simulink model "ALL_JP360_DBW_V6_5_1103"  (R2022a)
settings: Solver=FixedStepAuto  StartTime=0.0  StopTime=inf  FixedStep=0.01  RelTol=1e-3  EnableMultiTasking=on
model workspace (MAT data in the model file):
  g = 9.8
undefined symbols (not defined in the file or in its folder): canChannel, delta_v_p, IPM_Line_C0, IPM_Line_C1, IPM_Line_C2, IPM_Line_C3, M, M_p, MRR_ObjDistX, MRR_ObjDistY, MRR_ObjFusionCamID, MRR_ObjFusionSig, MRR_ObjID, MRR_ObjRelVelX, MRR_ObjRelVelY, MRR_ObjType, MRR_ObjUpdFlg, none, obj_vaild, untracktime, V, videoinput
libraries: canfdmsglib x230, canfdlib x76, slpidlib x24, simulink x18, dspstat3 x14, ctrlSharedLib x1, simulink_extras x1, imaqlib x1, realtime_pacer_lib x1, dspvision x1, visionsinks x1
(part 43 of 55)

== system ALL_JP360_DBW_V6_5_1103/MsgFromCAN/VR_ADCU_MsgFromCAN/VR_ADCU_IPM_Obj_04_0x653 ==
  VR_ADCU_IPM_Obj_04_0x653FromInData : Inport  OutDataTypeStr=Bus:CAN_FD_MESSAGE_BUS
  Bus Creator : BusCreator  Inputs=18  OutDataTypeStr=Bus:VR_ADCU_IPM_Obj_04_0x653  NonVirtualBus=on
  CAN FD Unpack : canfdmsglib/CAN FD Unpack  CANdbFile=HiFire_T360_P789_1R1V_Pri_Matrix_CAN_V2.3_20220810.dbc  MsgList=(none)  MsgName=IPM_Obj_04_0x653  ProtocolMode=CAN FD  MsgIDType=Standard (11-bit identifier)  MsgIdentifier=1619  MsgLength=32  SignalInfo={'IPM_ObjBlockCounter_04','13','11','BE','unsigned','Standard','0','1','0','0','2047';'IPM_ObjDistX_04','58','12','BE','unsigned','Standard','0','0.0625','0','0','254.9375';'IPM_ObjDistY_04','76','14','BE','unsigned','Standard','0','0.0078125','-64','-64','63.9922';'IPM_ObjID_04','16','8','BE','unsigned','Standard','0','1','0','0','255';'IPM_ObjRelAccelX_04','104','10','BE','unsigned','Standard','0','0.03125','-16','-16','15.9688';'IPM_ObjRelAccelY_04','126','10','BE','unsigned','Standard','0','0.03125','-16','-16','15.9688';'IPM_ObjRelVelX_04','95','13','BE','unsigned','Standard','0','0.03125','-128','-128','127.9688';'IPM_ObjRelVelY_04','98','13','BE','unsigned','Standard','0','0.03125','-128','-128','127.9688';'IPM_ObjType_04','54','4','BE','unsigned','Standard','0','1','0','0','15';'IPM_Obj_04_Checksum','248','16','BE','unsigned','Standard','0','1','0','0','65535';'IPM_Obj_04_MsgCounter','232','4','BE','unsigned','Standard','0','1','0','0','15';'IPM_Object_Age_04','37','11','BE','unsigned','Standard','0','1','0','0','2047';'IPM_Object_Existence_Probability_04','42','6','BE','unsigned','Standard','0','2','0','0','100';'IPM_Object_Heading_04','132','10','BE','unsigned','Standard','0','0.01','-3.14','-3.14','3.14';'IPM_Object_Height_04','167','9','BE','unsigned','Standard','0','0.01','0','0','5.11';'IPM_Object_Length_04','139','9','BE','unsigned','Standard','0','0.05','0','0','25.5';'IPM_Object_Motion_Status_04','161','3','BE','unsigned','Standard','0','1','0','0','7';'IPM_Object_Width_04','144','11','BE','unsigned','Standard','0','0.01','0','0','12'}  IDPort=off  TimestampPort=off  ErrorPort=off  RemotePort=off  LengthPort=off  StatusPort=off  BRSPort=off  ESIPort=off  DLCPort=off  ApplyMinMax=off
      settings: SourceProductBaseCode=ME,XP,VN  DataFormat=CANdb specified signals
  Data Type Conversion1 : DataTypeConversion  OutDataTypeStr=int16  SaturateOnIntegerOverflow=off  RndMeth=Floor
  Data Type Conversion10 : DataTypeConversion  OutDataTypeStr=uint16  SaturateOnIntegerOverflow=off  RndMeth=Floor
  Data Type Conversion{9,11,13,17} (4 alike) : DataTypeConversion  OutDataTypeStr=int8  SaturateOnIntegerOverflow=off  RndMeth=Floor
  Data Type Conversion12 : DataTypeConversion  OutDataTypeStr=int16  SaturateOnIntegerOverflow=off  RndMeth=Floor
  Data Type Conversion{2..3,5..8,14..16,18} (10 alike) : DataTypeConversion  OutDataTypeStr=single  SaturateOnIntegerOverflow=off  RndMeth=Floor
  Data Type Conversion4 : DataTypeConversion  OutDataTypeStr=uint8  SaturateOnIntegerOverflow=off  RndMeth=Floor
  VR_ADCU_IPM_Obj_04_0x653FromOutData : Outport  OutDataTypeStr=Bus:VR_ADCU_IPM_Obj_04_0x653
  wires:
  CAN FD Unpack/1 -> Data Type Conversion1/1
  CAN FD Unpack/2 -> Data Type Conversion2/1
  CAN FD Unpack/3 -> Data Type Conversion3/1
  CAN FD Unpack/4 -> Data Type Conversion4/1
  CAN FD Unpack/5 -> Data Type Conversion5/1
  CAN FD Unpack/6 -> Data Type Conversion6/1
  CAN FD Unpack/7 -> Data Type Conversion7/1
  CAN FD Unpack/8 -> Data Type Conversion8/1
  CAN FD Unpack/9 -> Data Type Conversion9/1
  CAN FD Unpack/10 -> Data Type Conversion10/1
  CAN FD Unpack/11 -> Data Type Conversion11/1
  CAN FD Unpack/12 -> Data Type Conversion12/1
  CAN FD Unpack/13 -> Data Type Conversion13/1
  CAN FD Unpack/14 -> Data Type Conversion14/1
  CAN FD Unpack/15 -> Data Type Conversion15/1
  CAN FD Unpack/16 -> Data Type Conversion16/1
  CAN FD Unpack/17 -> Data Type Conversion17/1
  CAN FD Unpack/18 -> Data Type Conversion18/1
  Data Type Conversion1/1 -> Bus Creator/1  "IPM_ObjBlockCounter_04"
  Data Type Conversion2/1 -> Bus Creator/2  "IPM_ObjDistX_04"
  Data Type Conversion3/1 -> Bus Creator/3  "IPM_ObjDistY_04"
  Data Type Conversion4/1 -> Bus Creator/4  "IPM_ObjID_04"
  Data Type Conversion5/1 -> Bus Creator/5  "IPM_ObjRelAccelX_04"
  Data Type Conversion6/1 -> Bus Creator/6  "IPM_ObjRelAccelY_04"
  Data Type Conversion7/1 -> Bus Creator/7  "IPM_ObjRelVelX_04"
  Data Type Conversion8/1 -> Bus Creator/8  "IPM_ObjRelVelY_04"
  Data Type Conversion9/1 -> Bus Creator/9  "IPM_ObjType_04"
  Data Type Conversion10/1 -> Bus Creator/10  "IPM_Obj_04_Checksum"
  Data Type Conversion11/1 -> Bus Creator/11  "IPM_Obj_04_MsgCounter"
  Data Type Conversion12/1 -> Bus Creator/12  "IPM_Object_Age_04"
  Data Type Conversion13/1 -> Bus Creator/13  "IPM_Object_Existence_Probability_04"
  Data Type Conversion14/1 -> Bus Creator/14  "IPM_Object_Heading_04"
  Data Type Conversion15/1 -> Bus Creator/15  "IPM_Object_Height_04"
  Data Type Conversion16/1 -> Bus Creator/16  "IPM_Object_Length_04"
  Data Type Conversion17/1 -> Bus Creator/17  "IPM_Object_Motion_Status_04"
  Data Type Conversion18/1 -> Bus Creator/18  "IPM_Object_Width_04"
  Bus Creator/1 -> VR_ADCU_IPM_Obj_04_0x653FromOutData/1  "VR_ADCU_IPM_Obj_04_0x653FromOutData"
  VR_ADCU_IPM_Obj_04_0x653FromInData/1 -> CAN FD Unpack/1  "VR_ADCU_IPM_Obj_04_0x653FromInData"

== system ALL_JP360_DBW_V6_5_1103/MsgFromCAN/VR_ADCU_MsgFromCAN/VR_ADCU_IPM_Obj_05_0x654 ==
  VR_ADCU_IPM_Obj_05_0x654FromInData : Inport  OutDataTypeStr=Bus:CAN_FD_MESSAGE_BUS
  Bus Creator : BusCreator  Inputs=18  OutDataTypeStr=Bus:VR_ADCU_IPM_Obj_05_0x654  NonVirtualBus=on
  CAN FD Unpack : canfdmsglib/CAN FD Unpack  CANdbFile=HiFire_T360_P789_1R1V_Pri_Matrix_CAN_V2.3_20220810.dbc  MsgList=(none)  MsgName=IPM_Obj_05_0x654  ProtocolMode=CAN FD  MsgIDType=Standard (11-bit identifier)  MsgIdentifier=1620  MsgLength=32  SignalInfo={'IPM_ObjBlockCounter_05','13','11','BE','unsigned','Standard','0','1','0','0','2047';'IPM_ObjDistX_05','58','12','BE','unsigned','Standard','0','0.0625','0','0','254.9375';'IPM_ObjDistY_05','76','14','BE','unsigned','Standard','0','0.0078125','-64','-64','63.9922';'IPM_ObjID_05','16','8','BE','unsigned','Standard','0','1','0','0','255';'IPM_ObjRelAccelX_05','104','10','BE','unsigned','Standard','0','0.03125','-16','-16','15.9688';'IPM_ObjRelAccelY_05','126','10','BE','unsigned','Standard','0','0.03125','-16','-16','15.9688';'IPM_ObjRelVelX_05','95','13','BE','unsigned','Standard','0','0.03125','-128','-128','127.9688';'IPM_ObjRelVelY_05','98','13','BE','unsigned','Standard','0','0.03125','-128','-128','127.9688';'IPM_ObjType_05','54','4','BE','unsigned','Standard','0','1','0','0','15';'IPM_Obj_05_Checksum','248','16','BE','unsigned','Standard','0','1','0','0','65535';'IPM_Obj_05_MsgCounter','232','4','BE','unsigned','Standard','0','1','0','0','15';'IPM_Object_Age_05','37','11','BE','unsigned','Standard','0','1','0','0','2047';'IPM_Object_Existence_Probability_05','42','6','BE','unsigned','Standard','0','2','0','0','100';'IPM_Object_Heading_05','132','10','BE','unsigned','Standard','0','0.01','-3.14','-3.14','3.14';'IPM_Object_Height_05','167','9','BE','unsigned','Standard','0','0.01','0','0','5.11';'IPM_Object_Length_05','139','9','BE','unsigned','Standard','0','0.05','0','0','25.5';'IPM_Object_Motion_Status_05','161','3','BE','unsigned','Standard','0','1','0','0','7';'IPM_Object_Width_05','144','11','BE','unsigned','Standard','0','0.01','0','0','12'}  IDPort=off  TimestampPort=off  ErrorPort=off  RemotePort=off  LengthPort=off  StatusPort=off  BRSPort=off  ESIPort=off  DLCPort=off  ApplyMinMax=off
      settings: SourceProductBaseCode=ME,XP,VN  DataFormat=CANdb specified signals
  Data Type Conversion1 : DataTypeConversion  OutDataTypeStr=int16  SaturateOnIntegerOverflow=off  RndMeth=Floor
  Data Type Conversion10 : DataTypeConversion  OutDataTypeStr=uint16  SaturateOnIntegerOverflow=off  RndMeth=Floor
  Data Type Conversion{9,11,13,17} (4 alike) : DataTypeConversion  OutDataTypeStr=int8  SaturateOnIntegerOverflow=off  RndMeth=Floor
  Data Type Conversion12 : DataTypeConversion  OutDataTypeStr=int16  SaturateOnIntegerOverflow=off  RndMeth=Floor
  Data Type Conversion{2..3,5..8,14..16,18} (10 alike) : DataTypeConversion  OutDataTypeStr=single  SaturateOnIntegerOverflow=off  RndMeth=Floor
  Data Type Conversion4 : DataTypeConversion  OutDataTypeStr=uint8  SaturateOnIntegerOverflow=off  RndMeth=Floor
  VR_ADCU_IPM_Obj_05_0x654FromOutData : Outport  OutDataTypeStr=Bus:VR_ADCU_IPM_Obj_05_0x654
  wires:
  CAN FD Unpack/1 -> Data Type Conversion1/1
  CAN FD Unpack/2 -> Data Type Conversion2/1
  CAN FD Unpack/3 -> Data Type Conversion3/1
  CAN FD Unpack/4 -> Data Type Conversion4/1
  CAN FD Unpack/5 -> Data Type Conversion5/1
  CAN FD Unpack/6 -> Data Type Conversion6/1
  CAN FD Unpack/7 -> Data Type Conversion7/1
  CAN FD Unpack/8 -> Data Type Conversion8/1
  CAN FD Unpack/9 -> Data Type Conversion9/1
  CAN FD Unpack/10 -> Data Type Conversion10/1
  CAN FD Unpack/11 -> Data Type Conversion11/1
  CAN FD Unpack/12 -> Data Type Conversion12/1
  CAN FD Unpack/13 -> Data Type Conversion13/1
  CAN FD Unpack/14 -> Data Type Conversion14/1
  CAN FD Unpack/15 -> Data Type Conversion15/1
  CAN FD Unpack/16 -> Data Type Conversion16/1
  CAN FD Unpack/17 -> Data Type Conversion17/1
  CAN FD Unpack/18 -> Data Type Conversion18/1
  Data Type Conversion1/1 -> Bus Creator/1  "IPM_ObjBlockCounter_05"
  Data Type Conversion2/1 -> Bus Creator/2  "IPM_ObjDistX_05"
  Data Type Conversion3/1 -> Bus Creator/3  "IPM_ObjDistY_05"
  Data Type Conversion4/1 -> Bus Creator/4  "IPM_ObjID_05"
  Data Type Conversion5/1 -> Bus Creator/5  "IPM_ObjRelAccelX_05"
  Data Type Conversion6/1 -> Bus Creator/6  "IPM_ObjRelAccelY_05"
  Data Type Conversion7/1 -> Bus Creator/7  "IPM_ObjRelVelX_05"
  Data Type Conversion8/1 -> Bus Creator/8  "IPM_ObjRelVelY_05"
  Data Type Conversion9/1 -> Bus Creator/9  "IPM_ObjType_05"
  Data Type Conversion10/1 -> Bus Creator/10  "IPM_Obj_05_Checksum"
  Data Type Conversion11/1 -> Bus Creator/11  "IPM_Obj_05_MsgCounter"
  Data Type Conversion12/1 -> Bus Creator/12  "IPM_Object_Age_05"
  Data Type Conversion13/1 -> Bus Creator/13  "IPM_Object_Existence_Probability_05"
  Data Type Conversion14/1 -> Bus Creator/14  "IPM_Object_Heading_05"
  Data Type Conversion15/1 -> Bus Creator/15  "IPM_Object_Height_05"
  Data Type Conversion16/1 -> Bus Creator/16  "IPM_Object_Length_05"
  Data Type Conversion17/1 -> Bus Creator/17  "IPM_Object_Motion_Status_05"
  Data Type Conversion18/1 -> Bus Creator/18  "IPM_Object_Width_05"
  Bus Creator/1 -> VR_ADCU_IPM_Obj_05_0x654FromOutData/1  "VR_ADCU_IPM_Obj_05_0x654FromOutData"
  VR_ADCU_IPM_Obj_05_0x654FromInData/1 -> CAN FD Unpack/1  "VR_ADCU_IPM_Obj_05_0x654FromInData"

== system ALL_JP360_DBW_V6_5_1103/MsgFromCAN/VR_ADCU_MsgFromCAN/VR_ADCU_IPM_Obj_06_0x655 ==
  VR_ADCU_IPM_Obj_06_0x655FromInData : Inport  OutDataTypeStr=Bus:CAN_FD_MESSAGE_BUS
  Bus Creator : BusCreator  Inputs=18  OutDataTypeStr=Bus:VR_ADCU_IPM_Obj_06_0x655  NonVirtualBus=on
  CAN FD Unpack : canfdmsglib/CAN FD Unpack  CANdbFile=HiFire_T360_P789_1R1V_Pri_Matrix_CAN_V2.3_20220810.dbc  MsgList=(none)  MsgName=IPM_Obj_06_0x655  ProtocolMode=CAN FD  MsgIDType=Standard (11-bit identifier)  MsgIdentifier=1621  MsgLength=32  SignalInfo={'IPM_ObjBlockCounter_06','13','11','BE','unsigned','Standard','0','1','0','0','2047';'IPM_ObjDistX_06','58','12','BE','unsigned','Standard','0','0.0625','0','0','254.9375';'IPM_ObjDistY_06','76','14','BE','unsigned','Standard','0','0.0078125','-64','-64','63.9922';'IPM_ObjID_06','16','8','BE','unsigned','Standard','0','1','0','0','255';'IPM_ObjRelAccelX_06','104','10','BE','unsigned','Standard','0','0.03125','-16','-16','15.9688';'IPM_ObjRelAccelY_06','126','10','BE','unsigned','Standard','0','0.03125','-16','-16','15.9688';'IPM_ObjRelVelX_06','95','13','BE','unsigned','Standard','0','0.03125','-128','-128','127.9688';'IPM_ObjRelVelY_06','98','13','BE','unsigned','Standard','0','0.03125','-128','-128','127.9688';'IPM_ObjType_06','54','4','BE','unsigned','Standard','0','1','0','0','15';'IPM_Obj_06_Checksum','248','16','BE','unsigned','Standard','0','1','0','0','65535';'IPM_Obj_06_MsgCounter','232','4','BE','unsigned','Standard','0','1','0','0','15';'IPM_Object_Age_06','37','11','BE','unsigned','Standard','0','1','0','0','2047';'IPM_Object_Existence_Probability_06','42','6','BE','unsigned','Standard','0','2','0','0','100';'IPM_Object_Heading_06','132','10','BE','unsigned','Standard','0','0.01','-3.14','-3.14','3.14';'IPM_Object_Height_06','167','9','BE','unsigned','Standard','0','0.01','0','0','5.11';'IPM_Object_Length_06','139','9','BE','unsigned','Standard','0','0.05','0','0','25.5';'IPM_Object_Motion_Status_06','161','3','BE','unsigned','Standard','0','1','0','0','7';'IPM_Object_Width_06','144','11','BE','unsigned','Standard','0','0.01','0','0','12'}  IDPort=off  TimestampPort=off  ErrorPort=off  RemotePort=off  LengthPort=off  StatusPort=off  BRSPort=off  ESIPort=off  DLCPort=off  ApplyMinMax=off
      settings: SourceProductBaseCode=ME,XP,VN  DataFormat=CANdb specified signals
  Data Type Conversion1 : DataTypeConversion  OutDataTypeStr=int16  SaturateOnIntegerOverflow=off  RndMeth=Floor
  Data Type Conversion10 : DataTypeConversion  OutDataTypeStr=uint16  SaturateOnIntegerOverflow=off  RndMeth=Floor
  Data Type Conversion{9,11,13,17} (4 alike) : DataTypeConversion  OutDataTypeStr=int8  SaturateOnIntegerOverflow=off  RndMeth=Floor
  Data Type Conversion12 : DataTypeConversion  OutDataTypeStr=int16  SaturateOnIntegerOverflow=off  RndMeth=Floor
  Data Type Conversion{2..3,5..8,14..16,18} (10 alike) : DataTypeConversion  OutDataTypeStr=single  SaturateOnIntegerOverflow=off  RndMeth=Floor
  Data Type Conversion4 : DataTypeConversion  OutDataTypeStr=uint8  SaturateOnIntegerOverflow=off  RndMeth=Floor
  VR_ADCU_IPM_Obj_06_0x655FromOutData : Outport  OutDataTypeStr=Bus:VR_ADCU_IPM_Obj_06_0x655
  wires:
  CAN FD Unpack/1 -> Data Type Conversion1/1
  CAN FD Unpack/2 -> Data Type Conversion2/1
  CAN FD Unpack/3 -> Data Type Conversion3/1
  CAN FD Unpack/4 -> Data Type Conversion4/1
  CAN FD Unpack/5 -> Data Type Conversion5/1
  CAN FD Unpack/6 -> Data Type Conversion6/1
  CAN FD Unpack/7 -> Data Type Conversion7/1
  CAN FD Unpack/8 -> Data Type Conversion8/1
  CAN FD Unpack/9 -> Data Type Conversion9/1
  CAN FD Unpack/10 -> Data Type Conversion10/1
  CAN FD Unpack/11 -> Data Type Conversion11/1
  CAN FD Unpack/12 -> Data Type Conversion12/1
  CAN FD Unpack/13 -> Data Type Conversion13/1
  CAN FD Unpack/14 -> Data Type Conversion14/1
  CAN FD Unpack/15 -> Data Type Conversion15/1
  CAN FD Unpack/16 -> Data Type Conversion16/1
  CAN FD Unpack/17 -> Data Type Conversion17/1
  CAN FD Unpack/18 -> Data Type Conversion18/1
  Data Type Conversion1/1 -> Bus Creator/1  "IPM_ObjBlockCounter_06"
  Data Type Conversion2/1 -> Bus Creator/2  "IPM_ObjDistX_06"
  Data Type Conversion3/1 -> Bus Creator/3  "IPM_ObjDistY_06"
  Data Type Conversion4/1 -> Bus Creator/4  "IPM_ObjID_06"
  Data Type Conversion5/1 -> Bus Creator/5  "IPM_ObjRelAccelX_06"
  Data Type Conversion6/1 -> Bus Creator/6  "IPM_ObjRelAccelY_06"
  Data Type Conversion7/1 -> Bus Creator/7  "IPM_ObjRelVelX_06"
  Data Type Conversion8/1 -> Bus Creator/8  "IPM_ObjRelVelY_06"
  Data Type Conversion9/1 -> Bus Creator/9  "IPM_ObjType_06"
  Data Type Conversion10/1 -> Bus Creator/10  "IPM_Obj_06_Checksum"
  Data Type Conversion11/1 -> Bus Creator/11  "IPM_Obj_06_MsgCounter"
  Data Type Conversion12/1 -> Bus Creator/12  "IPM_Object_Age_06"
  Data Type Conversion13/1 -> Bus Creator/13  "IPM_Object_Existence_Probability_06"
  Data Type Conversion14/1 -> Bus Creator/14  "IPM_Object_Heading_06"
  Data Type Conversion15/1 -> Bus Creator/15  "IPM_Object_Height_06"
  Data Type Conversion16/1 -> Bus Creator/16  "IPM_Object_Length_06"
  Data Type Conversion17/1 -> Bus Creator/17  "IPM_Object_Motion_Status_06"
  Data Type Conversion18/1 -> Bus Creator/18  "IPM_Object_Width_06"
  Bus Creator/1 -> VR_ADCU_IPM_Obj_06_0x655FromOutData/1  "VR_ADCU_IPM_Obj_06_0x655FromOutData"
  VR_ADCU_IPM_Obj_06_0x655FromInData/1 -> CAN FD Unpack/1  "VR_ADCU_IPM_Obj_06_0x655FromInData"

== system ALL_JP360_DBW_V6_5_1103/MsgFromCAN/VR_ADCU_MsgFromCAN/VR_ADCU_IPM_Obj_07_0x656 ==
  VR_ADCU_IPM_Obj_07_0x656FromInData : Inport  OutDataTypeStr=Bus:CAN_FD_MESSAGE_BUS
  Bus Creator : BusCreator  Inputs=18  OutDataTypeStr=Bus:VR_ADCU_IPM_Obj_07_0x656  NonVirtualBus=on
  CAN FD Unpack : canfdmsglib/CAN FD Unpack  CANdbFile=HiFire_T360_P789_1R1V_Pri_Matrix_CAN_V2.3_20220810.dbc  MsgList=(none)  MsgName=IPM_Obj_07_0x656  ProtocolMode=CAN FD  MsgIDType=Standard (11-bit identifier)  MsgIdentifier=1622  MsgLength=32  SignalInfo={'IPM_ObjBlockCounter_07','13','11','BE','unsigned','Standard','0','1','0','0','2047';'IPM_ObjDistX_07','58','12','BE','unsigned','Standard','0','0.0625','0','0','254.9375';'IPM_ObjDistY_07','76','14','BE','unsigned','Standard','0','0.0078125','-64','-64','63.9922';'IPM_ObjID_07','16','8','BE','unsigned','Standard','0','1','0','0','255';'IPM_ObjRelAccelX_07','104','10','BE','unsigned','Standard','0','0.03125','-16','-16','15.9688';'IPM_ObjRelAccelY_07','126','10','BE','unsigned','Standard','0','0.03125','-16','-16','15.9688';'IPM_ObjRelVelX_07','95','13','BE','unsigned','Standard','0','0.03125','-128','-128','127.9688';'IPM_ObjRelVelY_07','98','13','BE','unsigned','Standard','0','0.03125','-128','-128','127.9688';'IPM_ObjType_07','54','4','BE','unsigned','Standard','0','1','0','0','15';'IPM_Obj_07_Checksum','248','16','BE','unsigned','Standard','0','1','0','0','65535';'IPM_Obj_07_MsgCounter','232','4','BE','unsigned','Standard','0','1','0','0','15';'IPM_Object_Age_07','37','11','BE','unsigned','Standard','0','1','0','0','2047';'IPM_Object_Existence_Probability_07','42','6','BE','unsigned','Standard','0','2','0','0','100';'IPM_Object_Heading_07','132','10','BE','unsigned','Standard','0','0.01','-3.14','-3.14','3.14';'IPM_Object_Height_07','167','9','BE','unsigned','Standard','0','0.01','0','0','5.11';'IPM_Object_Length_07','139','9','BE','unsigned','Standard','0','0.05','0','0','25.5';'IPM_Object_Motion_Status_07','161','3','BE','unsigned','Standard','0','1','0','0','7';'IPM_Object_Width_07','144','11','BE','unsigned','Standard','0','0.01','0','0','12'}  IDPort=off  TimestampPort=off  ErrorPort=off  RemotePort=off  LengthPort=off  StatusPort=off  BRSPort=off  ESIPort=off  DLCPort=off  ApplyMinMax=off
      settings: SourceProductBaseCode=ME,XP,VN  DataFormat=CANdb specified signals
  Data Type Conversion1 : DataTypeConversion  OutDataTypeStr=int16  SaturateOnIntegerOverflow=off  RndMeth=Floor
  Data Type Conversion10 : DataTypeConversion  OutDataTypeStr=uint16  SaturateOnIntegerOverflow=off  RndMeth=Floor
  Data Type Conversion{9,11,13,17} (4 alike) : DataTypeConversion  OutDataTypeStr=int8  SaturateOnIntegerOverflow=off  RndMeth=Floor
  Data Type Conversion12 : DataTypeConversion  OutDataTypeStr=int16  SaturateOnIntegerOverflow=off  RndMeth=Floor
  Data Type Conversion{2..3,5..8,14..16,18} (10 alike) : DataTypeConversion  OutDataTypeStr=single  SaturateOnIntegerOverflow=off  RndMeth=Floor
  Data Type Conversion4 : DataTypeConversion  OutDataTypeStr=uint8  SaturateOnIntegerOverflow=off  RndMeth=Floor
  VR_ADCU_IPM_Obj_07_0x656FromOutData : Outport  OutDataTypeStr=Bus:VR_ADCU_IPM_Obj_07_0x656
  wires:
  CAN FD Unpack/1 -> Data Type Conversion1/1
  CAN FD Unpack/2 -> Data Type Conversion2/1
  CAN FD Unpack/3 -> Data Type Conversion3/1
  CAN FD Unpack/4 -> Data Type Conversion4/1
  CAN FD Unpack/5 -> Data Type Conversion5/1
  CAN FD Unpack/6 -> Data Type Conversion6/1
  CAN FD Unpack/7 -> Data Type Conversion7/1
  CAN FD Unpack/8 -> Data Type Conversion8/1
  CAN FD Unpack/9 -> Data Type Conversion9/1
  CAN FD Unpack/10 -> Data Type Conversion10/1
  CAN FD Unpack/11 -> Data Type Conversion11/1
  CAN FD Unpack/12 -> Data Type Conversion12/1
  CAN FD Unpack/13 -> Data Type Conversion13/1
  CAN FD Unpack/14 -> Data Type Conversion14/1
  CAN FD Unpack/15 -> Data Type Conversion15/1
  CAN FD Unpack/16 -> Data Type Conversion16/1
  CAN FD Unpack/17 -> Data Type Conversion17/1
  CAN FD Unpack/18 -> Data Type Conversion18/1
  Data Type Conversion1/1 -> Bus Creator/1  "IPM_ObjBlockCounter_07"
  Data Type Conversion2/1 -> Bus Creator/2  "IPM_ObjDistX_07"
  Data Type Conversion3/1 -> Bus Creator/3  "IPM_ObjDistY_07"
  Data Type Conversion4/1 -> Bus Creator/4  "IPM_ObjID_07"
  Data Type Conversion5/1 -> Bus Creator/5  "IPM_ObjRelAccelX_07"
  Data Type Conversion6/1 -> Bus Creator/6  "IPM_ObjRelAccelY_07"
  Data Type Conversion7/1 -> Bus Creator/7  "IPM_ObjRelVelX_07"
  Data Type Conversion8/1 -> Bus Creator/8  "IPM_ObjRelVelY_07"
  Data Type Conversion9/1 -> Bus Creator/9  "IPM_ObjType_07"
  Data Type Conversion10/1 -> Bus Creator/10  "IPM_Obj_07_Checksum"
  Data Type Conversion11/1 -> Bus Creator/11  "IPM_Obj_07_MsgCounter"
  Data Type Conversion12/1 -> Bus Creator/12  "IPM_Object_Age_07"
  Data Type Conversion13/1 -> Bus Creator/13  "IPM_Object_Existence_Probability_07"
  Data Type Conversion14/1 -> Bus Creator/14  "IPM_Object_Heading_07"
  Data Type Conversion15/1 -> Bus Creator/15  "IPM_Object_Height_07"
  Data Type Conversion16/1 -> Bus Creator/16  "IPM_Object_Length_07"
  Data Type Conversion17/1 -> Bus Creator/17  "IPM_Object_Motion_Status_07"
  Data Type Conversion18/1 -> Bus Creator/18  "IPM_Object_Width_07"
  Bus Creator/1 -> VR_ADCU_IPM_Obj_07_0x656FromOutData/1  "VR_ADCU_IPM_Obj_07_0x656FromOutData"
  VR_ADCU_IPM_Obj_07_0x656FromInData/1 -> CAN FD Unpack/1  "VR_ADCU_IPM_Obj_07_0x656FromInData"

== system ALL_JP360_DBW_V6_5_1103/MsgFromCAN/VR_ADCU_MsgFromCAN/VR_ADCU_IPM_Obj_08_0x657 ==
  VR_ADCU_IPM_Obj_08_0x657FromInData : Inport  OutDataTypeStr=Bus:CAN_FD_MESSAGE_BUS
  Bus Creator : BusCreator  Inputs=18  OutDataTypeStr=Bus:VR_ADCU_IPM_Obj_08_0x657  NonVirtualBus=on
  CAN FD Unpack : canfdmsglib/CAN FD Unpack  CANdbFile=HiFire_T360_P789_1R1V_Pri_Matrix_CAN_V2.3_20220810.dbc  MsgList=(none)  MsgName=IPM_Obj_08_0x657  ProtocolMode=CAN FD  MsgIDType=Standard (11-bit identifier)  MsgIdentifier=1623  MsgLength=32  SignalInfo={'IPM_ObjBlockCounter_08','13','11','BE','unsigned','Standard','0','1','0','0','2047';'IPM_ObjDistX_08','58','12','BE','unsigned','Standard','0','0.0625','0','0','254.9375';'IPM_ObjDistY_08','76','14','BE','unsigned','Standard','0','0.0078125','-64','-64','63.9922';'IPM_ObjID_08','16','8','BE','unsigned','Standard','0','1','0','0','255';'IPM_ObjRelAccelX_08','104','10','BE','unsigned','Standard','0','0.03125','-16','-16','15.9688';'IPM_ObjRelAccelY_08','126','10','BE','unsigned','Standard','0','0.03125','-16','-16','15.9688';'IPM_ObjRelVelX_08','95','13','BE','unsigned','Standard','0','0.03125','-128','-128','127.9688';'IPM_ObjRelVelY_08','98','13','BE','unsigned','Standard','0','0.03125','-128','-128','127.9688';'IPM_ObjType_08','54','4','BE','unsigned','Standard','0','1','0','0','15';'IPM_Obj_08_Checksum','248','16','BE','unsigned','Standard','0','1','0','0','65535';'IPM_Obj_08_MsgCounter','232','4','BE','unsigned','Standard','0','1','0','0','15';'IPM_Object_Age_08','37','11','BE','unsigned','Standard','0','1','0','0','2047';'IPM_Object_Existence_Probability_08','42','6','BE','unsigned','Standard','0','2','0','0','100';'IPM_Object_Heading_08','132','10','BE','unsigned','Standard','0','0.01','-3.14','-3.14','3.14';'IPM_Object_Height_08','167','9','BE','unsigned','Standard','0','0.01','0','0','5.11';'IPM_Object_Length_08','139','9','BE','unsigned','Standard','0','0.05','0','0','25.5';'IPM_Object_Motion_Status_08','161','3','BE','unsigned','Standard','0','1','0','0','7';'IPM_Object_Width_08','144','11','BE','unsigned','Standard','0','0.01','0','0','12'}  IDPort=off  TimestampPort=off  ErrorPort=off  RemotePort=off  LengthPort=off  StatusPort=off  BRSPort=off  ESIPort=off  DLCPort=off  ApplyMinMax=off
      settings: SourceProductBaseCode=ME,XP,VN  DataFormat=CANdb specified signals
  Data Type Conversion1 : DataTypeConversion  OutDataTypeStr=int16  SaturateOnIntegerOverflow=off  RndMeth=Floor
  Data Type Conversion10 : DataTypeConversion  OutDataTypeStr=uint16  SaturateOnIntegerOverflow=off  RndMeth=Floor
  Data Type Conversion{9,11,13,17} (4 alike) : DataTypeConversion  OutDataTypeStr=int8  SaturateOnIntegerOverflow=off  RndMeth=Floor
  Data Type Conversion12 : DataTypeConversion  OutDataTypeStr=int16  SaturateOnIntegerOverflow=off  RndMeth=Floor
  Data Type Conversion{2..3,5..8,14..16,18} (10 alike) : DataTypeConversion  OutDataTypeStr=single  SaturateOnIntegerOverflow=off  RndMeth=Floor
  Data Type Conversion4 : DataTypeConversion  OutDataTypeStr=uint8  SaturateOnIntegerOverflow=off  RndMeth=Floor
  VR_ADCU_IPM_Obj_08_0x657FromOutData : Outport  OutDataTypeStr=Bus:VR_ADCU_IPM_Obj_08_0x657
  wires:
  CAN FD Unpack/1 -> Data Type Conversion1/1
  CAN FD Unpack/2 -> Data Type Conversion2/1
  CAN FD Unpack/3 -> Data Type Conversion3/1
  CAN FD Unpack/4 -> Data Type Conversion4/1
  CAN FD Unpack/5 -> Data Type Conversion5/1
  CAN FD Unpack/6 -> Data Type Conversion6/1
  CAN FD Unpack/7 -> Data Type Conversion7/1
  CAN FD Unpack/8 -> Data Type Conversion8/1
  CAN FD Unpack/9 -> Data Type Conversion9/1
  CAN FD Unpack/10 -> Data Type Conversion10/1
  CAN FD Unpack/11 -> Data Type Conversion11/1
  CAN FD Unpack/12 -> Data Type Conversion12/1
  CAN FD Unpack/13 -> Data Type Conversion13/1
  CAN FD Unpack/14 -> Data Type Conversion14/1
  CAN FD Unpack/15 -> Data Type Conversion15/1
  CAN FD Unpack/16 -> Data Type Conversion16/1
  CAN FD Unpack/17 -> Data Type Conversion17/1
  CAN FD Unpack/18 -> Data Type Conversion18/1
  Data Type Conversion1/1 -> Bus Creator/1  "IPM_ObjBlockCounter_08"
  Data Type Conversion2/1 -> Bus Creator/2  "IPM_ObjDistX_08"
  Data Type Conversion3/1 -> Bus Creator/3  "IPM_ObjDistY_08"
  Data Type Conversion4/1 -> Bus Creator/4  "IPM_ObjID_08"
  Data Type Conversion5/1 -> Bus Creator/5  "IPM_ObjRelAccelX_08"
  Data Type Conversion6/1 -> Bus Creator/6  "IPM_ObjRelAccelY_08"
  Data Type Conversion7/1 -> Bus Creator/7  "IPM_ObjRelVelX_08"
  Data Type Conversion8/1 -> Bus Creator/8  "IPM_ObjRelVelY_08"
  Data Type Conversion9/1 -> Bus Creator/9  "IPM_ObjType_08"
  Data Type Conversion10/1 -> Bus Creator/10  "IPM_Obj_08_Checksum"
  Data Type Conversion11/1 -> Bus Creator/11  "IPM_Obj_08_MsgCounter"
  Data Type Conversion12/1 -> Bus Creator/12  "IPM_Object_Age_08"
  Data Type Conversion13/1 -> Bus Creator/13  "IPM_Object_Existence_Probability_08"
  Data Type Conversion14/1 -> Bus Creator/14  "IPM_Object_Heading_08"
  Data Type Conversion15/1 -> Bus Creator/15  "IPM_Object_Height_08"
  Data Type Conversion16/1 -> Bus Creator/16  "IPM_Object_Length_08"
  Data Type Conversion17/1 -> Bus Creator/17  "IPM_Object_Motion_Status_08"
  Data Type Conversion18/1 -> Bus Creator/18  "IPM_Object_Width_08"
  Bus Creator/1 -> VR_ADCU_IPM_Obj_08_0x657FromOutData/1  "VR_ADCU_IPM_Obj_08_0x657FromOutData"
  VR_ADCU_IPM_Obj_08_0x657FromInData/1 -> CAN FD Unpack/1  "VR_ADCU_IPM_Obj_08_0x657FromInData"

== system ALL_JP360_DBW_V6_5_1103/MsgFromCAN/VR_ADCU_MsgFromCAN/VR_ADCU_IPM_Obj_09_0x658 ==
  VR_ADCU_IPM_Obj_09_0x658FromInData : Inport  OutDataTypeStr=Bus:CAN_FD_MESSAGE_BUS
  Bus Creator : BusCreator  Inputs=18  OutDataTypeStr=Bus:VR_ADCU_IPM_Obj_09_0x658  NonVirtualBus=on
  CAN FD Unpack : canfdmsglib/CAN FD Unpack  CANdbFile=HiFire_T360_P789_1R1V_Pri_Matrix_CAN_V2.3_20220810.dbc  MsgList=(none)  MsgName=IPM_Obj_09_0x658  ProtocolMode=CAN FD  MsgIDType=Standard (11-bit identifier)  MsgIdentifier=1624  MsgLength=32  SignalInfo={'IPM_ObjBlockCounter_09','13','11','BE','unsigned','Standard','0','1','0','0','2047';'IPM_ObjDistX_09','58','12','BE','unsigned','Standard','0','0.0625','0','0','254.9375';'IPM_ObjDistY_09','76','14','BE','unsigned','Standard','0','0.0078125','-64','-64','63.9922';'IPM_ObjID_09','16','8','BE','unsigned','Standard','0','1','0','0','255';'IPM_ObjRelAccelX_09','104','10','BE','unsigned','Standard','0','0.03125','-16','-16','15.9688';'IPM_ObjRelAccelY_09','126','10','BE','unsigned','Standard','0','0.03125','-16','-16','15.9688';'IPM_ObjRelVelX_09','95','13','BE','unsigned','Standard','0','0.03125','-128','-128','127.9688';'IPM_ObjRelVelY_09','98','13','BE','unsigned','Standard','0','0.03125','-128','-128','127.9688';'IPM_ObjType_09','54','4','BE','unsigned','Standard','0','1','0','0','15';'IPM_Obj_09_Checksum','248','16','BE','unsigned','Standard','0','1','0','0','65535';'IPM_Obj_09_MsgCounter','232','4','BE','unsigned','Standard','0','1','0','0','15';'IPM_Object_Age_09','37','11','BE','unsigned','Standard','0','1','0','0','2047';'IPM_Object_Existence_Probability_09','42','6','BE','unsigned','Standard','0','2','0','0','100';'IPM_Object_Heading_09','132','10','BE','unsigned','Standard','0','0.01','-3.14','-3.14','3.14';'IPM_Object_Height_09','167','9','BE','unsigned','Standard','0','0.01','0','0','5.11';'IPM_Object_Length_09','139','9','BE','unsigned','Standard','0','0.05','0','0','25.5';'IPM_Object_Motion_Status_09','161','3','BE','unsigned','Standard','0','1','0','0','7';'IPM_Object_Width_09','144','11','BE','unsigned','Standard','0','0.01','0','0','12'}  IDPort=off  TimestampPort=off  ErrorPort=off  RemotePort=off  LengthPort=off  StatusPort=off  BRSPort=off  ESIPort=off  DLCPort=off  ApplyMinMax=off
      settings: SourceProductBaseCode=ME,XP,VN  DataFormat=CANdb specified signals
  Data Type Conversion1 : DataTypeConversion  OutDataTypeStr=int16  SaturateOnIntegerOverflow=off  RndMeth=Floor
  Data Type Conversion10 : DataTypeConversion  OutDataTypeStr=uint16  SaturateOnIntegerOverflow=off  RndMeth=Floor
  Data Type Conversion{9,11,13,17} (4 alike) : DataTypeConversion  OutDataTypeStr=int8  SaturateOnIntegerOverflow=off  RndMeth=Floor
  Data Type Conversion12 : DataTypeConversion  OutDataTypeStr=int16  SaturateOnIntegerOverflow=off  RndMeth=Floor
  Data Type Conversion{2..3,5..8,14..16,18} (10 alike) : DataTypeConversion  OutDataTypeStr=single  SaturateOnIntegerOverflow=off  RndMeth=Floor
  Data Type Conversion4 : DataTypeConversion  OutDataTypeStr=uint8  SaturateOnIntegerOverflow=off  RndMeth=Floor
  VR_ADCU_IPM_Obj_09_0x658FromOutData : Outport  OutDataTypeStr=Bus:VR_ADCU_IPM_Obj_09_0x658
  wires:
  CAN FD Unpack/1 -> Data Type Conversion1/1
  CAN FD Unpack/2 -> Data Type Conversion2/1
  CAN FD Unpack/3 -> Data Type Conversion3/1
  CAN FD Unpack/4 -> Data Type Conversion4/1
  CAN FD Unpack/5 -> Data Type Conversion5/1
  CAN FD Unpack/6 -> Data Type Conversion6/1
  CAN FD Unpack/7 -> Data Type Conversion7/1
  CAN FD Unpack/8 -> Data Type Conversion8/1
  CAN FD Unpack/9 -> Data Type Conversion9/1
  CAN FD Unpack/10 -> Data Type Conversion10/1
  CAN FD Unpack/11 -> Data Type Conversion11/1
  CAN FD Unpack/12 -> Data Type Conversion12/1
  CAN FD Unpack/13 -> Data Type Conversion13/1
  CAN FD Unpack/14 -> Data Type Conversion14/1
  CAN FD Unpack/15 -> Data Type Conversion15/1
  CAN FD Unpack/16 -> Data Type Conversion16/1
  CAN FD Unpack/17 -> Data Type Conversion17/1
  CAN FD Unpack/18 -> Data Type Conversion18/1
  Data Type Conversion1/1 -> Bus Creator/1  "IPM_ObjBlockCounter_09"
  Data Type Conversion2/1 -> Bus Creator/2  "IPM_ObjDistX_09"
  Data Type Conversion3/1 -> Bus Creator/3  "IPM_ObjDistY_09"
  Data Type Conversion4/1 -> Bus Creator/4  "IPM_ObjID_09"
  Data Type Conversion5/1 -> Bus Creator/5  "IPM_ObjRelAccelX_09"
  Data Type Conversion6/1 -> Bus Creator/6  "IPM_ObjRelAccelY_09"
  Data Type Conversion7/1 -> Bus Creator/7  "IPM_ObjRelVelX_09"
  Data Type Conversion8/1 -> Bus Creator/8  "IPM_ObjRelVelY_09"
  Data Type Conversion9/1 -> Bus Creator/9  "IPM_ObjType_09"
  Data Type Conversion10/1 -> Bus Creator/10  "IPM_Obj_09_Checksum"
  Data Type Conversion11/1 -> Bus Creator/11  "IPM_Obj_09_MsgCounter"
  Data Type Conversion12/1 -> Bus Creator/12  "IPM_Object_Age_09"
  Data Type Conversion13/1 -> Bus Creator/13  "IPM_Object_Existence_Probability_09"
  Data Type Conversion14/1 -> Bus Creator/14  "IPM_Object_Heading_09"
  Data Type Conversion15/1 -> Bus Creator/15  "IPM_Object_Height_09"
  Data Type Conversion16/1 -> Bus Creator/16  "IPM_Object_Length_09"
  Data Type Conversion17/1 -> Bus Creator/17  "IPM_Object_Motion_Status_09"
  Data Type Conversion18/1 -> Bus Creator/18  "IPM_Object_Width_09"
  Bus Creator/1 -> VR_ADCU_IPM_Obj_09_0x658FromOutData/1  "VR_ADCU_IPM_Obj_09_0x658FromOutData"
  VR_ADCU_IPM_Obj_09_0x658FromInData/1 -> CAN FD Unpack/1  "VR_ADCU_IPM_Obj_09_0x658FromInData"

== system ALL_JP360_DBW_V6_5_1103/MsgFromCAN/VR_ADCU_MsgFromCAN/VR_ADCU_IPM_Obj_10_0x659 ==
  VR_ADCU_IPM_Obj_10_0x659FromInData : Inport  OutDataTypeStr=Bus:CAN_FD_MESSAGE_BUS
  Bus Creator : BusCreator  Inputs=18  OutDataTypeStr=Bus:VR_ADCU_IPM_Obj_10_0x659  NonVirtualBus=on
  CAN FD Unpack : canfdmsglib/CAN FD Unpack  CANdbFile=HiFire_T360_P789_1R1V_Pri_Matrix_CAN_V2.3_20220810.dbc  MsgList=(none)  MsgName=IPM_Obj_10_0x659  ProtocolMode=CAN FD  MsgIDType=Standard (11-bit identifier)  MsgIdentifier=1625  MsgLength=32  SignalInfo={'IPM_ObjBlockCounter_10','13','11','BE','unsigned','Standard','0','1','0','0','2047';'IPM_ObjDistX_10','58','12','BE','unsigned','Standard','0','0.0625','0','0','254.9375';'IPM_ObjDistY_10','76','14','BE','unsigned','Standard','0','0.0078125','-64','-64','63.9922';'IPM_ObjID_10','16','8','BE','unsigned','Standard','0','1','0','0','255';'IPM_ObjRelAccelX_10','104','10','BE','unsigned','Standard','0','0.03125','-16','-16','15.9688';'IPM_ObjRelAccelY_10','126','10','BE','unsigned','Standard','0','0.03125','-16','-16','15.9688';'IPM_ObjRelVelX_10','95','13','BE','unsigned','Standard','0','0.03125','-128','-128','127.9688';'IPM_ObjRelVelY_10','98','13','BE','unsigned','Standard','0','0.03125','-128','-128','127.9688';'IPM_ObjType_10','54','4','BE','unsigned','Standard','0','1','0','0','15';'IPM_Obj_10_Checksum','248','16','BE','unsigned','Standard','0','1','0','0','65535';'IPM_Obj_10_MsgCounter','232','4','BE','unsigned','Standard','0','1','0','0','15';'IPM_Object_Age_10','37','11','BE','unsigned','Standard','0','1','0','0','2047';'IPM_Object_Existence_Probability_10','42','6','BE','unsigned','Standard','0','2','0','0','100';'IPM_Object_Heading_10','132','10','BE','unsigned','Standard','0','0.01','-3.14','-3.14','3.14';'IPM_Object_Height_10','167','9','BE','unsigned','Standard','0','0.01','0','0','5.11';'IPM_Object_Length_10','139','9','BE','unsigned','Standard','0','0.05','0','0','25.5';'IPM_Object_Motion_Status_10','161','3','BE','unsigned','Standard','0','1','0','0','7';'IPM_Object_Width_10','144','11','BE','unsigned','Standard','0','0.01','0','0','12'}  IDPort=off  TimestampPort=off  ErrorPort=off  RemotePort=off  LengthPort=off  StatusPort=off  BRSPort=off  ESIPort=off  DLCPort=off  ApplyMinMax=off
      settings: SourceProductBaseCode=ME,XP,VN  DataFormat=CANdb specified signals
  Data Type Conversion1 : DataTypeConversion  OutDataTypeStr=int16  SaturateOnIntegerOverflow=off  RndMeth=Floor
  Data Type Conversion10 : DataTypeConversion  OutDataTypeStr=uint16  SaturateOnIntegerOverflow=off  RndMeth=Floor
  Data Type Conversion{9,11,13,17} (4 alike) : DataTypeConversion  OutDataTypeStr=int8  SaturateOnIntegerOverflow=off  RndMeth=Floor
  Data Type Conversion12 : DataTypeConversion  OutDataTypeStr=int16  SaturateOnIntegerOverflow=off  RndMeth=Floor
  Data Type Conversion{2..3,5..8,14..16,18} (10 alike) : DataTypeConversion  OutDataTypeStr=single  SaturateOnIntegerOverflow=off  RndMeth=Floor
  Data Type Conversion4 : DataTypeConversion  OutDataTypeStr=uint8  SaturateOnIntegerOverflow=off  RndMeth=Floor
  VR_ADCU_IPM_Obj_10_0x659FromOutData : Outport  OutDataTypeStr=Bus:VR_ADCU_IPM_Obj_10_0x659
  wires:
  CAN FD Unpack/1 -> Data Type Conversion1/1
  CAN FD Unpack/2 -> Data Type Conversion2/1
  CAN FD Unpack/3 -> Data Type Conversion3/1
  CAN FD Unpack/4 -> Data Type Conversion4/1
  CAN FD Unpack/5 -> Data Type Conversion5/1
  CAN FD Unpack/6 -> Data Type Conversion6/1
  CAN FD Unpack/7 -> Data Type Conversion7/1
  CAN FD Unpack/8 -> Data Type Conversion8/1
  CAN FD Unpack/9 -> Data Type Conversion9/1
  CAN FD Unpack/10 -> Data Type Conversion10/1
  CAN FD Unpack/11 -> Data Type Conversion11/1
  CAN FD Unpack/12 -> Data Type Conversion12/1
  CAN FD Unpack/13 -> Data Type Conversion13/1
  CAN FD Unpack/14 -> Data Type Conversion14/1
  CAN FD Unpack/15 -> Data Type Conversion15/1
  CAN FD Unpack/16 -> Data Type Conversion16/1
  CAN FD Unpack/17 -> Data Type Conversion17/1
  CAN FD Unpack/18 -> Data Type Conversion18/1
  Data Type Conversion1/1 -> Bus Creator/1  "IPM_ObjBlockCounter_10"
  Data Type Conversion2/1 -> Bus Creator/2  "IPM_ObjDistX_10"
  Data Type Conversion3/1 -> Bus Creator/3  "IPM_ObjDistY_10"
  Data Type Conversion4/1 -> Bus Creator/4  "IPM_ObjID_10"
  Data Type Conversion5/1 -> Bus Creator/5  "IPM_ObjRelAccelX_10"
  Data Type Conversion6/1 -> Bus Creator/6  "IPM_ObjRelAccelY_10"
  Data Type Conversion7/1 -> Bus Creator/7  "IPM_ObjRelVelX_10"
  Data Type Conversion8/1 -> Bus Creator/8  "IPM_ObjRelVelY_10"
  Data Type Conversion9/1 -> Bus Creator/9  "IPM_ObjType_10"
  Data Type Conversion10/1 -> Bus Creator/10  "IPM_Obj_10_Checksum"
  Data Type Conversion11/1 -> Bus Creator/11  "IPM_Obj_10_MsgCounter"
  Data Type Conversion12/1 -> Bus Creator/12  "IPM_Object_Age_10"
  Data Type Conversion13/1 -> Bus Creator/13  "IPM_Object_Existence_Probability_10"
  Data Type Conversion14/1 -> Bus Creator/14  "IPM_Object_Heading_10"
  Data Type Conversion15/1 -> Bus Creator/15  "IPM_Object_Height_10"
  Data Type Conversion16/1 -> Bus Creator/16  "IPM_Object_Length_10"
  Data Type Conversion17/1 -> Bus Creator/17  "IPM_Object_Motion_Status_10"
  Data Type Conversion18/1 -> Bus Creator/18  "IPM_Object_Width_10"
  Bus Creator/1 -> VR_ADCU_IPM_Obj_10_0x659FromOutData/1  "VR_ADCU_IPM_Obj_10_0x659FromOutData"
  VR_ADCU_IPM_Obj_10_0x659FromInData/1 -> CAN FD Unpack/1  "VR_ADCU_IPM_Obj_10_0x659FromInData"

== system ALL_JP360_DBW_V6_5_1103/MsgFromCAN/VR_ADCU_MsgFromCAN/VR_ADCU_IPM_Obj_11_0x65A ==
  VR_ADCU_IPM_Obj_11_0x65AFromInData : Inport  OutDataTypeStr=Bus:CAN_FD_MESSAGE_BUS
  Bus Creator : BusCreator  Inputs=18  OutDataTypeStr=Bus:VR_ADCU_IPM_Obj_11_0x65A  NonVirtualBus=on
  CAN FD Unpack : canfdmsglib/CAN FD Unpack  CANdbFile=HiFire_T360_P789_1R1V_Pri_Matrix_CAN_V2.3_20220810.dbc  MsgList=(none)  MsgName=IPM_Obj_11_0x65A  ProtocolMode=CAN FD  MsgIDType=Standard (11-bit identifier)  MsgIdentifier=1626  MsgLength=32  SignalInfo={'IPM_ObjBlockCounter_11','13','11','BE','unsigned','Standard','0','1','0','0','2047';'IPM_ObjDistX_11','58','12','BE','unsigned','Standard','0','0.0625','0','0','254.9375';'IPM_ObjDistY_11','76','14','BE','unsigned','Standard','0','0.0078125','-64','-64','63.9922';'IPM_ObjID_11','16','8','BE','unsigned','Standard','0','1','0','0','255';'IPM_ObjRelAccelX_11','104','10','BE','unsigned','Standard','0','0.03125','-16','-16','15.9688';'IPM_ObjRelAccelY_11','126','10','BE','unsigned','Standard','0','0.03125','-16','-16','15.9688';'IPM_ObjRelVelX_11','95','13','BE','unsigned','Standard','0','0.03125','-128','-128','127.9688';'IPM_ObjRelVelY_11','98','13','BE','unsigned','Standard','0','0.03125','-128','-128','127.9688';'IPM_ObjType_11','54','4','BE','unsigned','Standard','0','1','0','0','15';'IPM_Obj_11_Checksum','248','16','BE','unsigned','Standard','0','1','0','0','65535';'IPM_Obj_11_MsgCounter','232','4','BE','unsigned','Standard','0','1','0','0','15';'IPM_Object_Age_11','37','11','BE','unsigned','Standard','0','1','0','0','2047';'IPM_Object_Existence_Probability_11','42','6','BE','unsigned','Standard','0','2','0','0','100';'IPM_Object_Heading_11','132','10','BE','unsigned','Standard','0','0.01','-3.14','-3.14','3.14';'IPM_Object_Height_11','167','9','BE','unsigned','Standard','0','0.01','0','0','5.11';'IPM_Object_Length_11','139','9','BE','unsigned','Standard','0','0.05','0','0','25.5';'IPM_Object_Motion_Status_11','161','3','BE','unsigned','Standard','0','1','0','0','7';'IPM_Object_Width_11','144','11','BE','unsigned','Standard','0','0.01','0','0','12'}  IDPort=off  TimestampPort=off  ErrorPort=off  RemotePort=off  LengthPort=off  StatusPort=off  BRSPort=off  ESIPort=off  DLCPort=off  ApplyMinMax=off
      settings: SourceProductBaseCode=ME,XP,VN  DataFormat=CANdb specified signals
  Data Type Conversion1 : DataTypeConversion  OutDataTypeStr=int16  SaturateOnIntegerOverflow=off  RndMeth=Floor
  Data Type Conversion10 : DataTypeConversion  OutDataTypeStr=uint16  SaturateOnIntegerOverflow=off  RndMeth=Floor
  Data Type Conversion{9,11,13,17} (4 alike) : DataTypeConversion  OutDataTypeStr=int8  SaturateOnIntegerOverflow=off  RndMeth=Floor
  Data Type Conversion12 : DataTypeConversion  OutDataTypeStr=int16  SaturateOnIntegerOverflow=off  RndMeth=Floor
  Data Type Conversion{2..3,5..8,14..16,18} (10 alike) : DataTypeConversion  OutDataTypeStr=single  SaturateOnIntegerOverflow=off  RndMeth=Floor
  Data Type Conversion4 : DataTypeConversion  OutDataTypeStr=uint8  SaturateOnIntegerOverflow=off  RndMeth=Floor
  VR_ADCU_IPM_Obj_11_0x65AFromOutData : Outport  OutDataTypeStr=Bus:VR_ADCU_IPM_Obj_11_0x65A
  wires:
  CAN FD Unpack/1 -> Data Type Conversion1/1
  CAN FD Unpack/2 -> Data Type Conversion2/1
  CAN FD Unpack/3 -> Data Type Conversion3/1
  CAN FD Unpack/4 -> Data Type Conversion4/1
  CAN FD Unpack/5 -> Data Type Conversion5/1
  CAN FD Unpack/6 -> Data Type Conversion6/1
  CAN FD Unpack/7 -> Data Type Conversion7/1
  CAN FD Unpack/8 -> Data Type Conversion8/1
  CAN FD Unpack/9 -> Data Type Conversion9/1
  CAN FD Unpack/10 -> Data Type Conversion10/1
  CAN FD Unpack/11 -> Data Type Conversion11/1
  CAN FD Unpack/12 -> Data Type Conversion12/1
  CAN FD Unpack/13 -> Data Type Conversion13/1
  CAN FD Unpack/14 -> Data Type Conversion14/1
  CAN FD Unpack/15 -> Data Type Conversion15/1
  CAN FD Unpack/16 -> Data Type Conversion16/1
  CAN FD Unpack/17 -> Data Type Conversion17/1
  CAN FD Unpack/18 -> Data Type Conversion18/1
  Data Type Conversion1/1 -> Bus Creator/1  "IPM_ObjBlockCounter_11"
  Data Type Conversion2/1 -> Bus Creator/2  "IPM_ObjDistX_11"
  Data Type Conversion3/1 -> Bus Creator/3  "IPM_ObjDistY_11"
  Data Type Conversion4/1 -> Bus Creator/4  "IPM_ObjID_11"
  Data Type Conversion5/1 -> Bus Creator/5  "IPM_ObjRelAccelX_11"
  Data Type Conversion6/1 -> Bus Creator/6  "IPM_ObjRelAccelY_11"
  Data Type Conversion7/1 -> Bus Creator/7  "IPM_ObjRelVelX_11"
  Data Type Conversion8/1 -> Bus Creator/8  "IPM_ObjRelVelY_11"
  Data Type Conversion9/1 -> Bus Creator/9  "IPM_ObjType_11"
  Data Type Conversion10/1 -> Bus Creator/10  "IPM_Obj_11_Checksum"
  Data Type Conversion11/1 -> Bus Creator/11  "IPM_Obj_11_MsgCounter"
  Data Type Conversion12/1 -> Bus Creator/12  "IPM_Object_Age_11"
  Data Type Conversion13/1 -> Bus Creator/13  "IPM_Object_Existence_Probability_11"
  Data Type Conversion14/1 -> Bus Creator/14  "IPM_Object_Heading_11"
  Data Type Conversion15/1 -> Bus Creator/15  "IPM_Object_Height_11"
  Data Type Conversion16/1 -> Bus Creator/16  "IPM_Object_Length_11"
  Data Type Conversion17/1 -> Bus Creator/17  "IPM_Object_Motion_Status_11"
  Data Type Conversion18/1 -> Bus Creator/18  "IPM_Object_Width_11"
  Bus Creator/1 -> VR_ADCU_IPM_Obj_11_0x65AFromOutData/1  "VR_ADCU_IPM_Obj_11_0x65AFromOutData"
  VR_ADCU_IPM_Obj_11_0x65AFromInData/1 -> CAN FD Unpack/1  "VR_ADCU_IPM_Obj_11_0x65AFromInData"

== system ALL_JP360_DBW_V6_5_1103/MsgFromCAN/VR_ADCU_MsgFromCAN/VR_ADCU_IPM_Obj_12_0x65B ==
  VR_ADCU_IPM_Obj_12_0x65BFromInData : Inport  OutDataTypeStr=Bus:CAN_FD_MESSAGE_BUS
  Bus Creator : BusCreator  Inputs=18  OutDataTypeStr=Bus:VR_ADCU_IPM_Obj_12_0x65B  NonVirtualBus=on
  CAN FD Unpack : canfdmsglib/CAN FD Unpack  CANdbFile=HiFire_T360_P789_1R1V_Pri_Matrix_CAN_V2.3_20220810.dbc  MsgList=(none)  MsgName=IPM_Obj_12_0x65B  ProtocolMode=CAN FD  MsgIDType=Standard (11-bit identifier)  MsgIdentifier=1627  MsgLength=32  SignalInfo={'IPM_ObjBlockCounter_12','13','11','BE','unsigned','Standard','0','1','0','0','2047';'IPM_ObjDistX_12','58','12','BE','unsigned','Standard','0','0.0625','0','0','254.9375';'IPM_ObjDistY_12','76','14','BE','unsigned','Standard','0','0.0078125','-64','-64','63.9922';'IPM_ObjID_12','16','8','BE','unsigned','Standard','0','1','0','0','255';'IPM_ObjRelAccelX_12','104','10','BE','unsigned','Standard','0','0.03125','-16','-16','15.9688';'IPM_ObjRelAccelY_12','126','10','BE','unsigned','Standard','0','0.03125','-16','-16','15.9688';'IPM_ObjRelVelX_12','95','13','BE','unsigned','Standard','0','0.03125','-128','-128','127.9688';'IPM_ObjRelVelY_12','98','13','BE','unsigned','Standard','0','0.03125','-128','-128','127.9688';'IPM_ObjType_12','54','4','BE','unsigned','Standard','0','1','0','0','15';'IPM_Obj_12_Checksum','248','16','BE','unsigned','Standard','0','1','0','0','65535';'IPM_Obj_12_MsgCounter','232','4','BE','unsigned','Standard','0','1','0','0','15';'IPM_Object_Age_12','37','11','BE','unsigned','Standard','0','1','0','0','2047';'IPM_Object_Existence_Probability_12','42','6','BE','unsigned','Standard','0','2','0','0','100';'IPM_Object_Heading_12','132','10','BE','unsigned','Standard','0','0.01','-3.14','-3.14','3.14';'IPM_Object_Height_12','167','9','BE','unsigned','Standard','0','0.01','0','0','5.11';'IPM_Object_Length_12','139','9','BE','unsigned','Standard','0','0.05','0','0','25.5';'IPM_Object_Motion_Status_12','161','3','BE','unsigned','Standard','0','1','0','0','7';'IPM_Object_Width_12','144','11','BE','unsigned','Standard','0','0.01','0','0','12'}  IDPort=off  TimestampPort=off  ErrorPort=off  RemotePort=off  LengthPort=off  StatusPort=off  BRSPort=off  ESIPort=off  DLCPort=off  ApplyMinMax=off
      settings: SourceProductBaseCode=ME,XP,VN  DataFormat=CANdb specified signals
  Data Type Conversion1 : DataTypeConversion  OutDataTypeStr=int16  SaturateOnIntegerOverflow=off  RndMeth=Floor
  Data Type Conversion10 : DataTypeConversion  OutDataTypeStr=uint16  SaturateOnIntegerOverflow=off  RndMeth=Floor
  Data Type Conversion{9,11,13,17} (4 alike) : DataTypeConversion  OutDataTypeStr=int8  SaturateOnIntegerOverflow=off  RndMeth=Floor
  Data Type Conversion12 : DataTypeConversion  OutDataTypeStr=int16  SaturateOnIntegerOverflow=off  RndMeth=Floor
  Data Type Conversion{2..3,5..8,14..16,18} (10 alike) : DataTypeConversion  OutDataTypeStr=single  SaturateOnIntegerOverflow=off  RndMeth=Floor
  Data Type Conversion4 : DataTypeConversion  OutDataTypeStr=uint8  SaturateOnIntegerOverflow=off  RndMeth=Floor
  VR_ADCU_IPM_Obj_12_0x65BFromOutData : Outport  OutDataTypeStr=Bus:VR_ADCU_IPM_Obj_12_0x65B
  wires:
  CAN FD Unpack/1 -> Data Type Conversion1/1
  CAN FD Unpack/2 -> Data Type Conversion2/1
  CAN FD Unpack/3 -> Data Type Conversion3/1
  CAN FD Unpack/4 -> Data Type Conversion4/1
  CAN FD Unpack/5 -> Data Type Conversion5/1
  CAN FD Unpack/6 -> Data Type Conversion6/1
  CAN FD Unpack/7 -> Data Type Conversion7/1
  CAN FD Unpack/8 -> Data Type Conversion8/1
  CAN FD Unpack/9 -> Data Type Conversion9/1
  CAN FD Unpack/10 -> Data Type Conversion10/1
  CAN FD Unpack/11 -> Data Type Conversion11/1
  CAN FD Unpack/12 -> Data Type Conversion12/1
  CAN FD Unpack/13 -> Data Type Conversion13/1
  CAN FD Unpack/14 -> Data Type Conversion14/1
  CAN FD Unpack/15 -> Data Type Conversion15/1
  CAN FD Unpack/16 -> Data Type Conversion16/1
  CAN FD Unpack/17 -> Data Type Conversion17/1
  CAN FD Unpack/18 -> Data Type Conversion18/1
  Data Type Conversion1/1 -> Bus Creator/1  "IPM_ObjBlockCounter_12"
  Data Type Conversion2/1 -> Bus Creator/2  "IPM_ObjDistX_12"
  Data Type Conversion3/1 -> Bus Creator/3  "IPM_ObjDistY_12"
  Data Type Conversion4/1 -> Bus Creator/4  "IPM_ObjID_12"
  Data Type Conversion5/1 -> Bus Creator/5  "IPM_ObjRelAccelX_12"
  Data Type Conversion6/1 -> Bus Creator/6  "IPM_ObjRelAccelY_12"
  Data Type Conversion7/1 -> Bus Creator/7  "IPM_ObjRelVelX_12"
  Data Type Conversion8/1 -> Bus Creator/8  "IPM_ObjRelVelY_12"
  Data Type Conversion9/1 -> Bus Creator/9  "IPM_ObjType_12"
  Data Type Conversion10/1 -> Bus Creator/10  "IPM_Obj_12_Checksum"
  Data Type Conversion11/1 -> Bus Creator/11  "IPM_Obj_12_MsgCounter"
  Data Type Conversion12/1 -> Bus Creator/12  "IPM_Object_Age_12"
  Data Type Conversion13/1 -> Bus Creator/13  "IPM_Object_Existence_Probability_12"
  Data Type Conversion14/1 -> Bus Creator/14  "IPM_Object_Heading_12"
  Data Type Conversion15/1 -> Bus Creator/15  "IPM_Object_Height_12"
  Data Type Conversion16/1 -> Bus Creator/16  "IPM_Object_Length_12"
  Data Type Conversion17/1 -> Bus Creator/17  "IPM_Object_Motion_Status_12"
  Data Type Conversion18/1 -> Bus Creator/18  "IPM_Object_Width_12"
  Bus Creator/1 -> VR_ADCU_IPM_Obj_12_0x65BFromOutData/1  "VR_ADCU_IPM_Obj_12_0x65BFromOutData"
  VR_ADCU_IPM_Obj_12_0x65BFromInData/1 -> CAN FD Unpack/1  "VR_ADCU_IPM_Obj_12_0x65BFromInData"
